simulink model "RR_Forces"  (R2023b)
settings: Solver=VariableStepAuto  StartTime=0.0  StopTime=200  RelTol=1e-3
values from neighbouring files (symbols this model uses):
  RR_Aero_Aoa = [-40 -20 -10 -5 0 5 10 20 40]    [RR.mat]    (also in aero.m = [-40.0, -20.0, -10.0, -5.0, 0.0, 5.0, 10.0, 20.0, 40.0])
  RR_Aero_CD = [0.682566420597 0.618503123563 0.559439658146 0.524132967178 0.485737326161 0.447874599784 0.410140259349 0.344355457301 0.271986762452 0.285740001736 0.220860646778 0.173194791928 ... (405 elements, 9x9x5)]    [RR.mat]    (also in aero.m = flip([0.271986762452 0.048967807354 0.024623797928 0.0311930)
  RR_Aero_CL = [-1.32787481318 -1.28000797148 -1.22978921447 -1.19580936529 -1.15925228344 -1.11732991534 -1.07321949156 -0.982213833372 -0.840672452343 -1.01110225062 -0.901800471345 -0.804191382013 ... (405 elements, 9x9x5)]    [RR.mat]    (also in aero.m = flip([-0.840672452343 -0.271053660865 0.064194032020 0.23384)
  RR_Aero_CMy = [0.261776710059 0.227892723507 0.194122810948 0.17203964717 0.149197278338 0.123782621534 0.09809104025 0.048156954183 -0.022673613914 0.230490752369 0.172298182326 0.122095577928 ... (405 elements, 9x9x5)]    [RR.mat]    (also in aero.m = flip([-0.022673613914 -0.123256713392 -0.153636001960 -0.164)
  RR_Aero_Elevons = [-40 -20 -10 -5 0 5 10 20 40]    [RR.mat]    (also in aero.m = [-40.0, -20.0, -10.0, -5.0, 0.0, 5.0, 10.0, 20.0, 40.0])
  RR_Aero_Mach = [0.01 0.1 0.2 0.5 0.9]    [RR.mat]    (also in aero.m = [0.01, 0.1, 0.2, 0.5, 0.9])
  RR_Iyy = 4.432    [RR.mat]
  RR_Motors_Thrust = [4.04656097579 98.9159349639]    [RR.mat]
  RR_Motors_Thrust_Alt_Lut = [0 10000 20000 30000]    [RR.mat]
  RR_Motors_Thrust_Pct_Lut = [1 0.705882352941 0.470588235294 0.352941176471]    [RR.mat]
  RR_Span = 3.6    [RR.mat]
  RR_X_CG = 0.732425    [RR.mat]
  RR_X_NP = 0.9170209    [RR.mat]
  SIM_ELEVONS = 0.155    [RR.mat]    (also in RR_Forces_ws.m; RR_Pitch_ws.m)
  SIM_G = 32.174    [RR.mat]    (also in RR_Forces_ws.m = G; RR_Pitch_ws.m = G; RR_Target_sim_ws.m = G; RR_Target_ws.m = G)
  SIM_INITAL_ALT = -1000    [RR.mat]    (also in RR_Forces_ws.m; RR_Pitch_ws.m = 0; RR_Target_sim_ws.m = 0; RR_Target_ws.m = 0)
  SIM_INITAL_VEL = 750    [RR.mat]    (also in RR_Forces_ws.m; RR_Pitch_ws.m = 11; RR_Target_sim_ws.m = 15; RR_Target_ws.m = 15)
  SIM_THROTTLE = 0.5    [RR.mat]    (also in RR_Forces_ws.m; RR_Pitch_ws.m = 1)
libraries: aerolibasang x2, simulink_extras x2, aerolib6dof2 x1, aerolibadyn x1, aerolibatmos2 x1
settings Model: Creator=jrighetti  LastModifiedBy=jrighetti

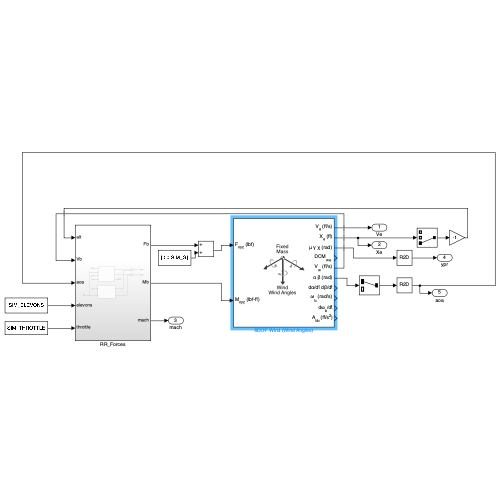
[thumbnail: Simulink's stored preview of the top-level diagram]
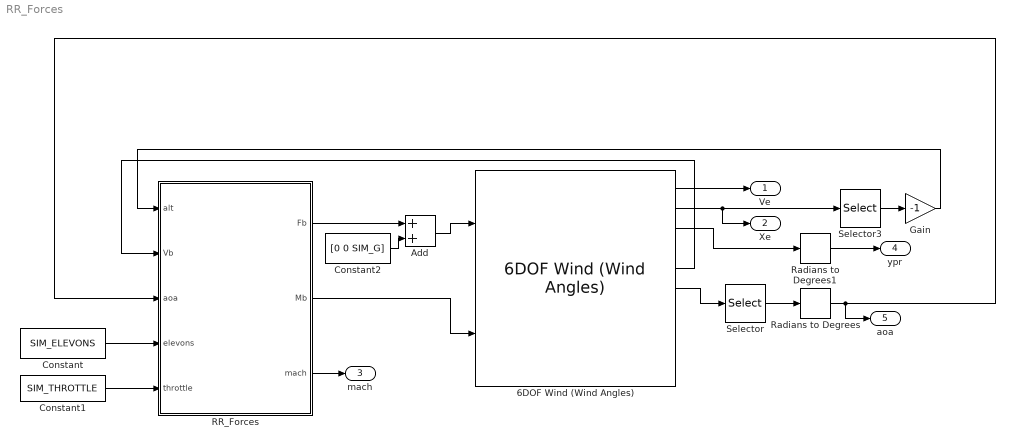
== system RR_Forces ==
  6DOF Wind (Wind Angles) : aerolib6dof2/6DOF Wind (Wind Angles)  units=English (Velocity in ft/s)  mtype=Fixed  rep=Wind Angles  xme_0=[0 0 SIM_INITAL_ALT]  Vm_0=[SIM_INITAL_VEL 0 0]  wind_0=[0 0 0]  pm_0=[0 0 0]  mass_0=RR_Total_Mass  mass_e=RR_Total_Mass  mass_f=RR_Total_Dry_Mass  inertia=diag([1 RR_Iyy 1])  inertia_e=diag([1 RR_Iyy 1])  inertia_f=diag([1 RR_Iyy 1])*0.75  vre_flag=on  abi_flag=off  xme_statename=''  Vm_statename=''  alpha_statename=''  beta_statename=''  wind_statename=''  quat_statename=''  pm_statename=''  mass_statename=''
  Add : Sum
  Constant : Constant  Value=SIM_ELEVONS
  Constant1 : Constant  Value=SIM_THROTTLE
  Constant2 : Constant  Value=[0 0 SIM_G]
  Gain : Gain  Gain=-1
  RR_Forces : Subsystem
  Radians to Degrees : simulink_extras/Transformations/Radians to Degrees
  Radians to Degrees1 : simulink_extras/Transformations/Radians to Degrees
  Selector : Selector  InputPortWidth=2  IndexOptions=Index vector (dialog)  Indices=1  OutputSizes=1
  Selector3 : Selector  InputPortWidth=3  IndexOptions=Index vector (dialog)  Indices=3  OutputSizes=1
  Ve : Outport
  Xe : Outport  Port=2
  mach : Outport  Port=3
  ypr : Outport  Port=4
  aoa : Outport  Port=5
  wires:
  6DOF Wind (Wind Angles)/2 -> Xe/1, Selector3/1
  Selector3/1 -> Gain/1
  Gain/1 -> RR_Forces/1(alt)
  6DOF Wind (Wind Angles)/5 -> RR_Forces/2(Vb)
  RR_Forces/1(Fb) -> Add/1
  RR_Forces/2(Mb) -> 6DOF Wind (Wind Angles)/2
  6DOF Wind (Wind Angles)/6 -> Selector/1
  Selector/1 -> Radians to Degrees/1
  Radians to Degrees/1 -> aoa/1, RR_Forces/3(aoa)
  6DOF Wind (Wind Angles)/1 -> Ve/1
  Constant/1 -> RR_Forces/4(elevons)
  Constant1/1 -> RR_Forces/5(throttle)
  RR_Forces/3(mach) -> mach/1
  6DOF Wind (Wind Angles)/3 -> Radians to Degrees1/1
  Add/1 -> 6DOF Wind (Wind Angles)/1
  Constant2/1 -> Add/2
  Radians to Degrees1/1 -> ypr/1

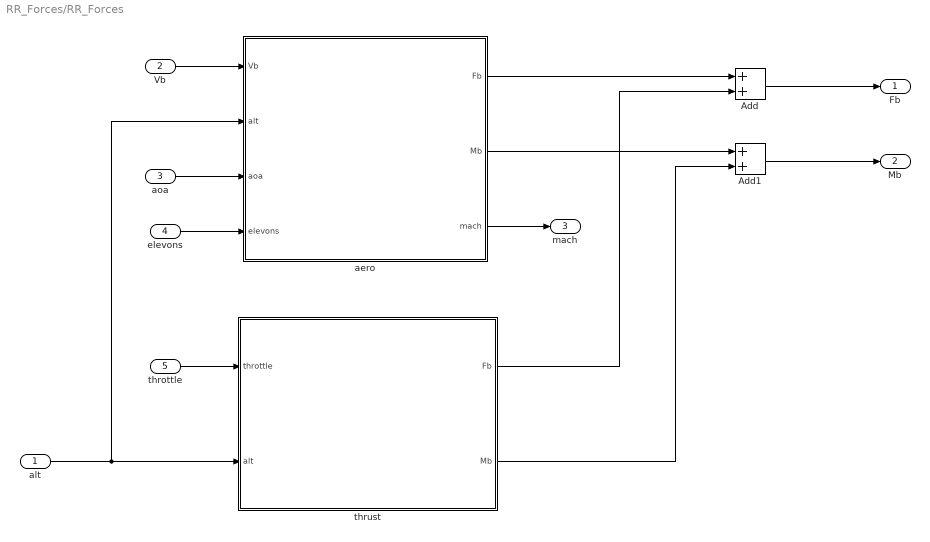
== system RR_Forces/RR_Forces ==
  alt : Inport
  Vb : Inport  Port=2
  aoa : Inport  Port=3
  elevons : Inport  Port=4
  throttle : Inport  Port=5
  Add : Sum
  Add1 : Sum
  aero : Subsystem
  thrust : Subsystem
  Fb : Outport
  Mb : Outport  Port=2
  mach : Outport  Port=3
  wires:
  alt/1 -> aero/2(alt), thrust/2(alt)
  Vb/1 -> aero/1(Vb)
  aoa/1 -> aero/3(aoa)
  elevons/1 -> aero/4(elevons)
  throttle/1 -> thrust/1(throttle)
  aero/1(Fb) -> Add/1
  thrust/1(Fb) -> Add/2
  Add/1 -> Fb/1
  aero/2(Mb) -> Add1/1
  thrust/2(Mb) -> Add1/2
  Add1/1 -> Mb/1
  aero/3(mach) -> mach/1

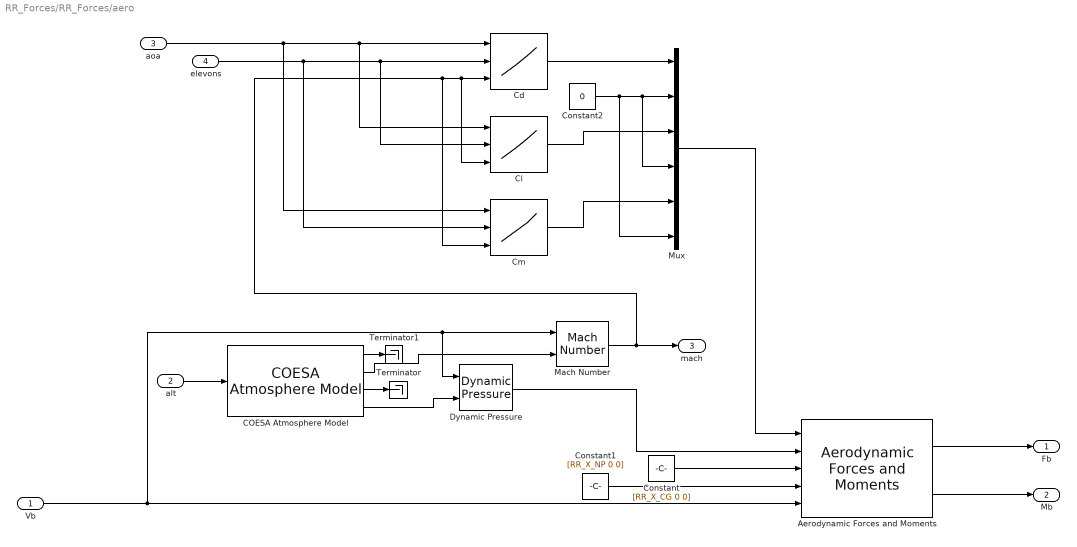
== system RR_Forces/RR_Forces/aero ==
  Vb : Inport
  alt : Inport  Port=2
  aoa : Inport  Port=3
  elevons : Inport  Port=4
  "Aerodynamic Forces and Moments " : aerolibadyn/Aerodynamic Forces and Moments   inputAxes=Wind  outputForceAxes=Body  outputMomentAxes=Body  S=RR_AERO_S  b=RR_Span  cbar=RR_AERO_CORD
  COESA Atmosphere Model : aerolibatmos2/COESA Atmosphere Model  units=English (Velocity in ft/s)  spec=1976 COESA-extended U.S. Standard Atmosphere  model=Profile  profile_var=High temperature  profile_percent=1%  profile_alt=5 km (16404 ft)  envelope_var=High temperature  envelope_percent=1%  action=Warning
  Cd : Lookup_n-D  NumberOfTableDimensions=3  BreakpointsForDimension1=RR_Aero_Aoa  BreakpointsForDimension2=RR_Aero_Elevons  BreakpointsForDimension3=RR_Aero_Mach  BreakpointsForDimension1DataTypeStr=Inherit: Inherit from 'Breakpoint data'  Table=RR_Aero_CD  TableDataTypeStr=Inherit: Inherit from 'Table data'  InternalRulePriority=Speed  RndMeth=Simplest
      settings: InputPortMap=u0,u1,u2
  Cl : Lookup_n-D  NumberOfTableDimensions=3  BreakpointsForDimension1=RR_Aero_Aoa  BreakpointsForDimension2=RR_Aero_Elevons  BreakpointsForDimension3=RR_Aero_Mach  Table=RR_Aero_CL  DiagnosticForOutOfRangeInput=Warning  InternalRulePriority=Speed  RndMeth=Simplest
      settings: InputPortMap=u0,u1,u2
  Cm : Lookup_n-D  NumberOfTableDimensions=3  BreakpointsForDimension1=RR_Aero_Aoa  BreakpointsForDimension2=RR_Aero_Elevons  BreakpointsForDimension3=RR_Aero_Mach  Table=RR_Aero_CMy  DiagnosticForOutOfRangeInput=Warning  InternalRulePriority=Speed  RndMeth=Simplest
      settings: InputPortMap=u0,u1,u2
  Constant : Constant  Value=[RR_X_CG 0 0]
  Constant1 : Constant  Value=[RR_X_NP 0 0]
  Constant2 : Constant  Value=0
  Dynamic Pressure : aerolibasang/Dynamic Pressure
  Mach Number : aerolibasang/Mach Number
  Mux : Mux  Inputs=6
  Terminator : Terminator
  Terminator1 : Terminator
  Fb : Outport
  Mb : Outport  Port=2
  mach : Outport  Port=3
  wires:
  Dynamic Pressure/1 -> "Aerodynamic Forces and Moments "/2
  Constant2/1 -> Mux/6, Mux/4, Mux/2
  alt/1 -> COESA Atmosphere Model/1
  "Aerodynamic Forces and Moments "/1 -> Fb/1
  COESA Atmosphere Model/2 -> Mach Number/2
  COESA Atmosphere Model/3 -> Terminator/1
  Constant/1 -> "Aerodynamic Forces and Moments "/3
  COESA Atmosphere Model/4 -> Dynamic Pressure/2
  "Aerodynamic Forces and Moments "/2 -> Mb/1
  elevons/1 -> Cm/2, Cl/2, Cd/2
  Mach Number/1 -> mach/1, Cm/3, Cl/3, Cd/3
  Mux/1 -> "Aerodynamic Forces and Moments "/1
  Cl/1 -> Mux/3
  Constant1/1 -> "Aerodynamic Forces and Moments "/4
  aoa/1 -> Cm/1, Cl/1, Cd/1
  Cd/1 -> Mux/1
  COESA Atmosphere Model/1 -> Terminator1/1
  Cm/1 -> Mux/5
  Vb/1 -> "Aerodynamic Forces and Moments "/5, Dynamic Pressure/1, Mach Number/1

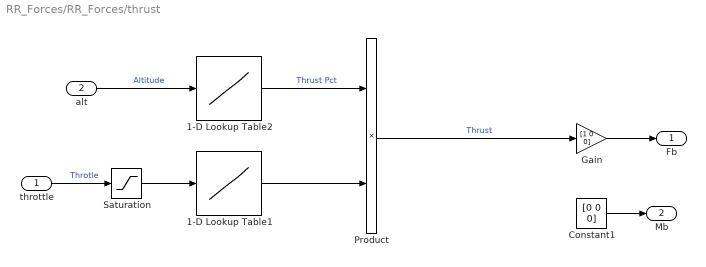
== system RR_Forces/RR_Forces/thrust ==
  throttle : Inport
  alt : Inport  Port=2
  1-D Lookup Table1 : Lookup_n-D  NumberOfTableDimensions=1  BreakpointsForDimension1=[0,1]  Table=RR_Motors_Thrust  InternalRulePriority=Speed  RndMeth=Simplest
  1-D Lookup Table2 : Lookup_n-D  NumberOfTableDimensions=1  BreakpointsForDimension1=RR_Motors_Thrust_Alt_Lut  Table=RR_Motors_Thrust_Pct_Lut  InternalRulePriority=Speed  RndMeth=Simplest
  Constant1 : Constant  Value=[0 0 0]
  Gain : Gain  Gain=[1 0 0]
  Product : Product
  Saturation : Saturate  UpperLimit=1.0  LowerLimit=0.0
  Fb : Outport
  Mb : Outport  Port=2
  wires:
  throttle/1 -> Saturation/1  "Throtle"
  alt/1 -> 1-D Lookup Table2/1  "Altitude"
  1-D Lookup Table2/1 -> Product/1  "Thrust Pct"
  1-D Lookup Table1/1 -> Product/2
  Saturation/1 -> 1-D Lookup Table1/1
  Product/1 -> Gain/1  "Thrust"
  Gain/1 -> Fb/1
  Constant1/1 -> Mb/1
